simulink model "gm_radarSim4"  (R2023b)
settings: Solver=FixedStepAuto  StartTime=0.0  StopTime=simTime  RelTol=1e-3
libraries: dspsrcs4 x3, dspstat3 x2, paullib x2, simulink x1
settings Model: Creator=pbroo  LastModifiedBy=pbroo
settings SolverCC: AutoInsertRateTranBlk=on
settings OptimizationCC: BlockReduction=off  ConditionallyExecuteInputs=off  DefaultParameterBehavior=Inlined
settings DebuggingCC: AlgebraicLoopMsg=error  InheritedTsInSrcMsg=none  SingleTaskRateTransMsg=error
settings HardwareCC: ProdBitPerPointer=32  ProdBitPerSizeT=32  ProdBitPerPtrDiffT=32  ProdLargestAtomicFloat=None  ProdIntDivRoundTo=Undefined  ProdEndianess=Unspecified  ProdWordSize=32  ProdHWDeviceType=ASIC/FPGA->ASIC/FPGA  TargetBitPerPointer=64  TargetBitPerSizeT=64  TargetBitPerPtrDiffT=64  TargetLongLongMode=on  TargetIntDivRoundTo=Zero  TargetEndianess=LittleEndian  TargetWordSize=64  TargetHWDeviceType=Custom Processor->MATLAB Host Computer  ProdEqTarget=off

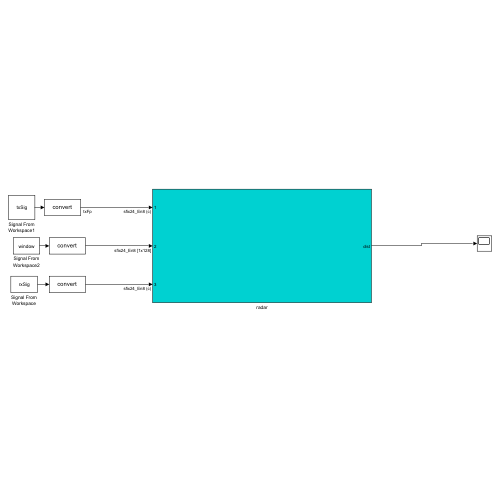
[thumbnail: Simulink's stored preview of the top-level diagram]
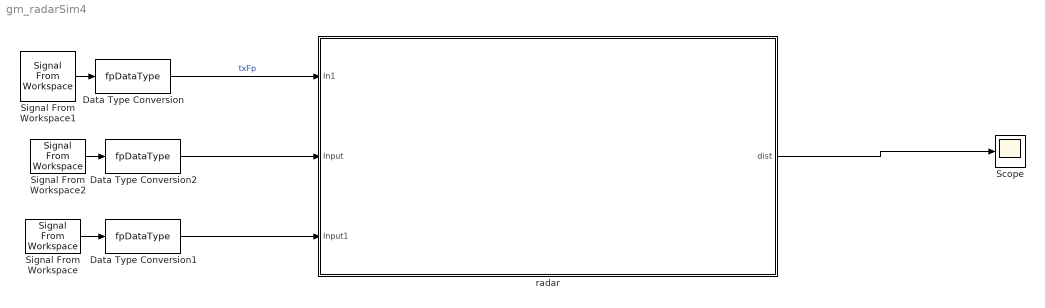
== system gm_radarSim4 ==
  Data Type Conversion : DataTypeConversion  OutDataTypeStr=fpDataType  SaturateOnIntegerOverflow=off  RndMeth=Floor
  Data Type Conversion1 : DataTypeConversion  OutDataTypeStr=fpDataType  SaturateOnIntegerOverflow=off  RndMeth=Floor
  Data Type Conversion2 : DataTypeConversion  OutDataTypeStr=fpDataType  SaturateOnIntegerOverflow=off  RndMeth=Floor
  Scope : Scope
  Signal From Workspace : dspsrcs4/Signal From Workspace  X=rxSig  Ts=1  nsamps=1  OutputAfterFinalValue=Setting to zero  ignoreOrWarnInputAndFrameLengths=off  OutputFrames=off
  Signal From Workspace1 : dspsrcs4/Signal From Workspace  X=txSig  Ts=1  nsamps=1  OutputAfterFinalValue=Setting to zero  ignoreOrWarnInputAndFrameLengths=off  OutputFrames=off
  Signal From Workspace2 : dspsrcs4/Signal From Workspace  X=window  Ts=1  nsamps=1  OutputAfterFinalValue=Setting to zero  ignoreOrWarnInputAndFrameLengths=off  OutputFrames=off
  radar : Subsystem
  wires:
  Data Type Conversion2/1 -> radar/2(Input)
  Signal From Workspace2/1 -> Data Type Conversion2/1
  Data Type Conversion1/1 -> radar/3(Input1)
  Data Type Conversion/1 -> radar/1(In1)  "txFp"
  radar/1(dist) -> Scope/1
  Signal From Workspace/1 -> Data Type Conversion1/1
  Signal From Workspace1/1 -> Data Type Conversion/1

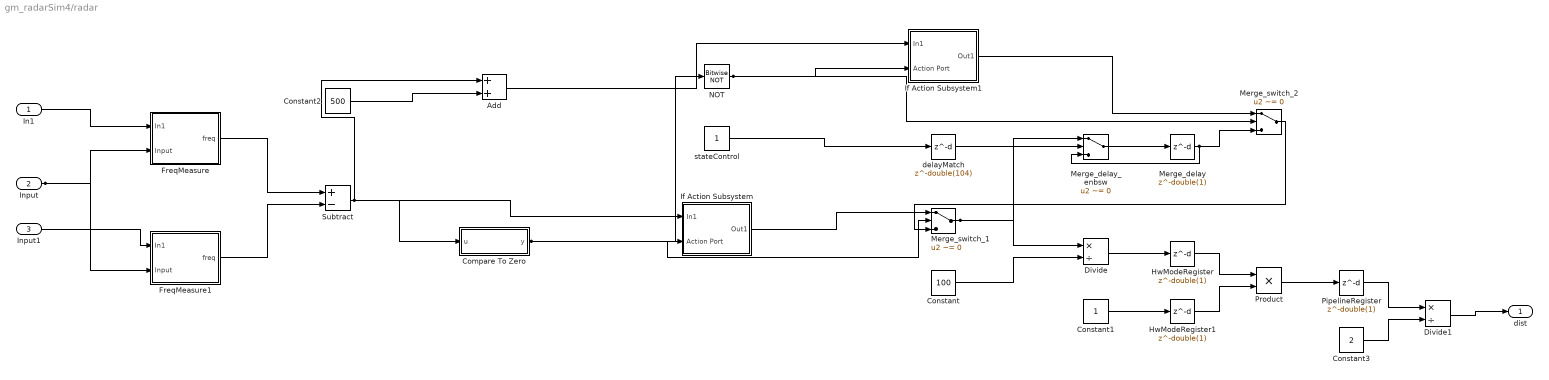
== system gm_radarSim4/radar ==
  In1 : Inport  OutDataTypeStr=fixdt(1, 24, 8)  PortDimensions=1  SampleTime=1
      settings: SignalType=complex
  Input : Inport  Port=2  OutDataTypeStr=fixdt(1, 24, 8)  PortDimensions=[1 128]  SampleTime=1
  Input1 : Inport  Port=3  OutDataTypeStr=fixdt(1, 24, 8)  PortDimensions=1  SampleTime=1
      settings: SignalType=complex
  Add : Sum  OutDataTypeStr=fixdt(1, 24, 8)  AccumDataTypeStr=fixdt(1, 25, 8)  SampleTime=1
  Compare To Zero : Subsystem  mask(Compare To Zero){relop=>=, OutDataTypeStr=boolean, ZeroCross=on}
      mask prompts: relop "Simulink:masks:Operator_MP"; OutDataTypeStr "Simulink:masks:OutputDataType_MP"; ZeroCross "Simulink:masks:EnableZerocrossingDetection_MP"
      mask help: Simulink:masks:CompareToZero_MD
      mask init:
      | OutDataTypeStr = 'boolean';
      | ZeroCross = 'on';
      | blkName = 'radarSim4/radar/Compare\nTo Zero';
      | relop = '>=';
      | setValue = 'boolean';
      mask TypeOptions relop: == | ~= | < | <= | >= | >
      mask TypeOptions OutDataTypeStr: Simulink:masks:uint8 | Simulink:masks:boolean
      mask Callback ZeroCross: sl('zeroCrossEnable', gcbh);
      mask Display: disp([relop,' 0'])
  Constant : Constant  Value=100  OutDataTypeStr=int16  SampleTime=1
  Constant1 : Constant  OutDataTypeStr=int16  SampleTime=1
  Constant2 : Constant  Value=500  OutDataTypeStr=fixdt(1, 24, 8)  SampleTime=1
  Constant3 : Constant  Value=2  VectorParams1D=off  OutDataTypeStr=int16  SampleTime=1
  Divide : Product  Inputs=*/  OutDataTypeStr=fixdt(1, 24, 8)  RndMeth=Simplest  SaturateOnIntegerOverflow=on  SampleTime=1
  Divide1 : Product  Inputs=*/  OutDataTypeStr=fixdt(1, 40, 8)  RndMeth=Simplest  SaturateOnIntegerOverflow=on  SampleTime=1
  FreqMeasure : Subsystem
  FreqMeasure1 : Subsystem
  HwModeRegister : Delay  DelayLength=double(1)  InitialCondition=0  SampleTime=1
  HwModeRegister1 : Delay  DelayLength=double(1)  InitialCondition=0  SampleTime=1
  If Action Subsystem : Subsystem
  If Action Subsystem1 : Subsystem
  Merge_delay : Delay  DelayLength=double(1)  InitialCondition=0  SampleTime=1
  Merge_delay_enbsw : Switch  Criteria=u2 ~= 0  Threshold=double(0)  OutDataTypeStr=fixdt(1, 24, 8)  SampleTime=1  SaturateOnIntegerOverflow=off  InputSameDT=off
  Merge_switch_1 : Switch  Criteria=u2 ~= 0  Threshold=double(0)  OutDataTypeStr=fixdt(1, 24, 8)  SampleTime=1  SaturateOnIntegerOverflow=off  InputSameDT=off
  Merge_switch_2 : Switch  Criteria=u2 ~= 0  Threshold=double(0)  OutDataTypeStr=fixdt(1, 24, 8)  SampleTime=1  SaturateOnIntegerOverflow=off  InputSameDT=off
  NOT : simulink/Logic and Bit Operations/Bitwise Operator  logicop=NOT  UseBitMask=off  BitMask=double(0)  BitMaskRealWorld=Real World Value
  PipelineRegister : Delay  DelayLength=double(1)  InitialCondition=0  SampleTime=1
  Product : Product  Inputs=**  OutDataTypeStr=fixdt(1, 40, 8)  SampleTime=1
  Subtract : Sum  Inputs=+-  OutDataTypeStr=fixdt(1, 24, 8)  AccumDataTypeStr=fixdt(1, 57, 0)  SampleTime=1
  delayMatch : Delay  DelayLength=double(104)  InitialCondition=0  SampleTime=1
  stateControl : Constant  OutDataTypeStr=boolean  SampleTime=1
  dist : Outport  SampleTime=1
  wires:
  In1/1 -> FreqMeasure/1(In1)
  Input/1 -> FreqMeasure1/2(Input), FreqMeasure/2(Input)
  Input1/1 -> FreqMeasure1/1(In1)
  Add/1 -> If Action Subsystem1/1(In1)
  Compare To Zero/1(y) -> NOT/1, If Action Subsystem/2(Action Port), Merge_switch_1/2
  Constant/1 -> Divide/2
  Constant1/1 -> HwModeRegister1/1
  Constant2/1 -> Add/2
  Constant3/1 -> Divide1/2
  Divide/1 -> HwModeRegister/1
  Divide1/1 -> dist/1
  FreqMeasure/1(freq) -> Subtract/1
  FreqMeasure1/1(freq) -> Subtract/2
  PipelineRegister/1 -> Divide1/1
  Subtract/1 -> Add/1, Compare To Zero/1(u), If Action Subsystem/1(In1)
  NOT/1 -> If Action Subsystem1/2(Action Port), Merge_switch_2/2
  stateControl/1 -> delayMatch/1
  Merge_switch_1/1 -> Merge_delay_enbsw/1, Divide/1
  delayMatch/1 -> Merge_delay_enbsw/2
  If Action Subsystem1/1(Out1) -> Merge_switch_2/1
  If Action Subsystem/1(Out1) -> Merge_switch_1/1
  Merge_switch_2/1 -> Merge_switch_1/3
  Merge_delay/1 -> Merge_delay_enbsw/3, Merge_switch_2/3
  Merge_delay_enbsw/1 -> Merge_delay/1
  Product/1 -> PipelineRegister/1
  HwModeRegister/1 -> Product/1
  HwModeRegister1/1 -> Product/2

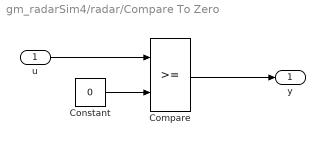
== system gm_radarSim4/radar/Compare To Zero ==
  u : Inport  OutDataTypeStr=fixdt(1, 24, 8)  SampleTime=1
  Compare : RelationalOperator  OutDataTypeStr=boolean
  Constant : Constant  DisableCoverage=on  Value=0  OutDataTypeStr=Inherit: Inherit via back propagation  SampleTime=-1  PreserveConstantTs=on
  y : Outport  SampleTime=1
  wires:
  u/1 -> Compare/1
  Compare/1 -> y/1
  Constant/1 -> Compare/2

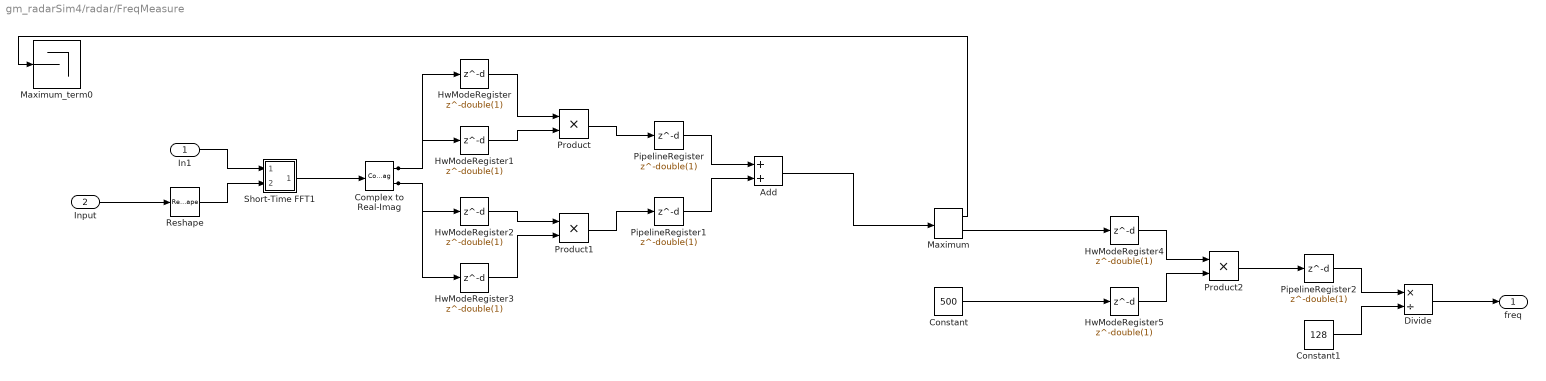
== system gm_radarSim4/radar/FreqMeasure ==
  In1 : Inport  OutDataTypeStr=fixdt(1, 24, 8)  PortDimensions=1  SampleTime=1
      settings: SignalType=complex
  Input : Inport  Port=2  OutDataTypeStr=fixdt(1, 24, 8)  PortDimensions=[1 128]  SampleTime=1
  Add : Sum  OutDataTypeStr=fixdt(1, 63, 16)  AccumDataTypeStr=fixdt(1, 63, 16)  SampleTime=1
  Complex to Real-Imag : ComplexToRealImag  SampleTime=1
  Constant : Constant  Value=500  OutDataTypeStr=fixdt(1, 24, 8)  SampleTime=1
  Constant1 : Constant  Value=128  OutDataTypeStr=fixdt(1, 24, 8)  SampleTime=1
  Divide : Product  Inputs=*/  OutDataTypeStr=fixdt(1, 56, 0)  RndMeth=Simplest  SaturateOnIntegerOverflow=on  SampleTime=1
  HwModeRegister{,1..5} (6 alike) : Delay  DelayLength=double(1)  InitialCondition=0  SampleTime=1
  Maximum : dspstat3/Maximum  operation=maximum  fcn=Value and Index  indexBase=One  operateOver=Each column  Dimension=1  InputProcessing=Columns as channels (frame based)  reset=None  roiEnable=off  roiType=Rectangles  roiPortion=Entire ROI  roiOutput=Individual statistics for each ROI  roiFlag=off  roundingMode=Floor  overflowMode=off  accumDataTypeStr=Inherit: Same as product output  accumLastDataTypeStr=Inherit: Same as product output
  Maximum_term0 : Terminator
  PipelineRegister : Delay  DelayLength=double(1)  InitialCondition=0  SampleTime=1
  PipelineRegister1 : Delay  DelayLength=double(1)  InitialCondition=0  SampleTime=1
  PipelineRegister2 : Delay  DelayLength=double(1)  InitialCondition=0  SampleTime=1
  Product : Product  Inputs=**  OutDataTypeStr=fixdt(1, 62, 16)  SampleTime=1
  Product1 : Product  Inputs=**  OutDataTypeStr=fixdt(1, 62, 16)  SampleTime=1
  Product2 : Product  Inputs=**  OutDataTypeStr=fixdt(1, 56, 8)  SampleTime=1
  Reshape : Reshape  OutputDimensionality=Column vector (2-D)
  Short-Time FFT1 : Subsystem
  freq : Outport  SampleTime=1
  wires:
  In1/1 -> Short-Time FFT1/1(In1)
  Input/1 -> Reshape/1
  Add/1 -> Maximum/1
  Complex to Real-Imag/1 -> HwModeRegister/1, HwModeRegister1/1
  Complex to Real-Imag/2 -> HwModeRegister2/1, HwModeRegister3/1
  Constant/1 -> HwModeRegister5/1
  Constant1/1 -> Divide/2
  Divide/1 -> freq/1
  Maximum/1 -> Maximum_term0/1
  Maximum/2 -> HwModeRegister4/1
  PipelineRegister/1 -> Add/1
  PipelineRegister1/1 -> Add/2
  PipelineRegister2/1 -> Divide/1
  Reshape/1 -> Short-Time FFT1/2(In2)
  Short-Time FFT1/1(Out1) -> Complex to Real-Imag/1
  Product/1 -> PipelineRegister/1
  HwModeRegister/1 -> Product/1
  HwModeRegister1/1 -> Product/2
  Product1/1 -> PipelineRegister1/1
  HwModeRegister2/1 -> Product1/1
  HwModeRegister3/1 -> Product1/2
  Product2/1 -> PipelineRegister2/1
  HwModeRegister4/1 -> Product2/1
  HwModeRegister5/1 -> Product2/2

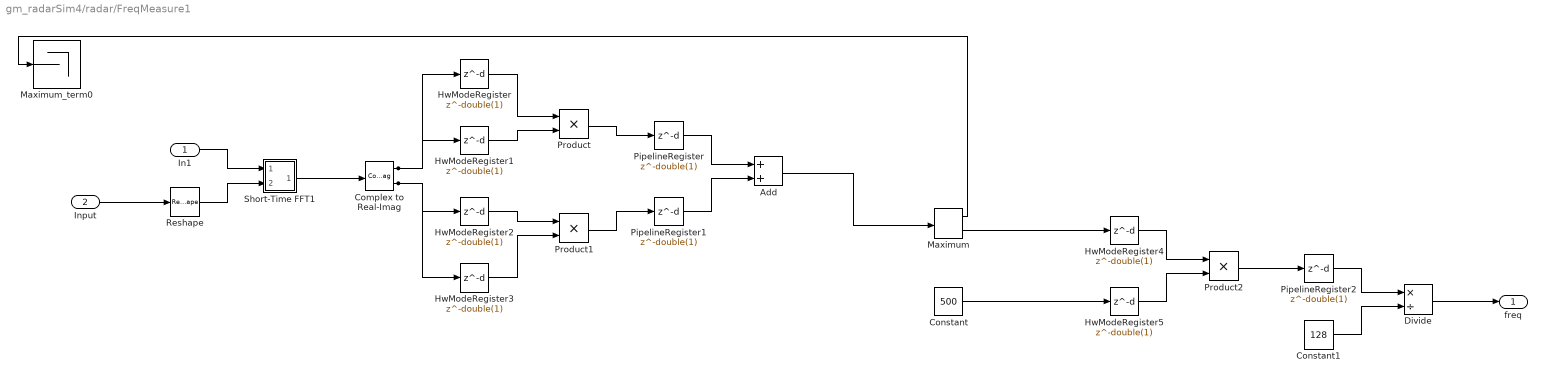
== system gm_radarSim4/radar/FreqMeasure1 ==
  In1 : Inport  OutDataTypeStr=fixdt(1, 24, 8)  PortDimensions=1  SampleTime=1
      settings: SignalType=complex
  Input : Inport  Port=2  OutDataTypeStr=fixdt(1, 24, 8)  PortDimensions=[1 128]  SampleTime=1
  Add : Sum  OutDataTypeStr=fixdt(1, 63, 16)  AccumDataTypeStr=fixdt(1, 63, 16)  SampleTime=1
  Complex to Real-Imag : ComplexToRealImag  SampleTime=1
  Constant : Constant  Value=500  OutDataTypeStr=fixdt(1, 24, 8)  SampleTime=1
  Constant1 : Constant  Value=128  OutDataTypeStr=fixdt(1, 24, 8)  SampleTime=1
  Divide : Product  Inputs=*/  OutDataTypeStr=fixdt(1, 56, 0)  RndMeth=Simplest  SaturateOnIntegerOverflow=on  SampleTime=1
  HwModeRegister{,1..5} (6 alike) : Delay  DelayLength=double(1)  InitialCondition=0  SampleTime=1
  Maximum : dspstat3/Maximum  operation=maximum  fcn=Value and Index  indexBase=One  operateOver=Each column  Dimension=1  InputProcessing=Columns as channels (frame based)  reset=None  roiEnable=off  roiType=Rectangles  roiPortion=Entire ROI  roiOutput=Individual statistics for each ROI  roiFlag=off  roundingMode=Floor  overflowMode=off  accumDataTypeStr=Inherit: Same as product output  accumLastDataTypeStr=Inherit: Same as product output
  Maximum_term0 : Terminator
  PipelineRegister : Delay  DelayLength=double(1)  InitialCondition=0  SampleTime=1
  PipelineRegister1 : Delay  DelayLength=double(1)  InitialCondition=0  SampleTime=1
  PipelineRegister2 : Delay  DelayLength=double(1)  InitialCondition=0  SampleTime=1
  Product : Product  Inputs=**  OutDataTypeStr=fixdt(1, 62, 16)  SampleTime=1
  Product1 : Product  Inputs=**  OutDataTypeStr=fixdt(1, 62, 16)  SampleTime=1
  Product2 : Product  Inputs=**  OutDataTypeStr=fixdt(1, 56, 8)  SampleTime=1
  Reshape : Reshape  OutputDimensionality=Column vector (2-D)
  Short-Time FFT1 : Subsystem
  freq : Outport  SampleTime=1
  wires:
  In1/1 -> Short-Time FFT1/1(In1)
  Input/1 -> Reshape/1
  Add/1 -> Maximum/1
  Complex to Real-Imag/1 -> HwModeRegister/1, HwModeRegister1/1
  Complex to Real-Imag/2 -> HwModeRegister2/1, HwModeRegister3/1
  Constant/1 -> HwModeRegister5/1
  Constant1/1 -> Divide/2
  Divide/1 -> freq/1
  Maximum/1 -> Maximum_term0/1
  Maximum/2 -> HwModeRegister4/1
  PipelineRegister/1 -> Add/1
  PipelineRegister1/1 -> Add/2
  PipelineRegister2/1 -> Divide/1
  Reshape/1 -> Short-Time FFT1/2(In2)
  Short-Time FFT1/1(Out1) -> Complex to Real-Imag/1
  Product/1 -> PipelineRegister/1
  HwModeRegister/1 -> Product/1
  HwModeRegister1/1 -> Product/2
  Product1/1 -> PipelineRegister1/1
  HwModeRegister2/1 -> Product1/1
  HwModeRegister3/1 -> Product1/2
  Product2/1 -> PipelineRegister2/1
  HwModeRegister4/1 -> Product2/1
  HwModeRegister5/1 -> Product2/2

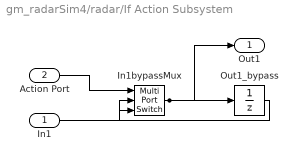
== system gm_radarSim4/radar/If Action Subsystem ==
  In1 : Inport  OutDataTypeStr=fixdt(1, 24, 8)  PortDimensions=1  SampleTime=1
  Action Port : Inport  Port=2  OutDataTypeStr=boolean  SampleTime=1
  In1bypassMux : MultiPortSwitch  DataPortOrder=Zero-based contiguous  Inputs=2  zeroidx=on  OutDataTypeStr=fixdt(1, 24, 8)  SampleTime=1  SaturateOnIntegerOverflow=off  InputSameDT=off
  Out1_bypass : UnitDelay  InitialCondition="fi(0,1,24,8,\"hex\",\"000000\")"  SampleTime=1
  Out1 : Outport  SampleTime=1  InitialOutput=0
  wires:
  In1bypassMux/1 -> Out1/1, Out1_bypass/1
  Action Port/1 -> In1bypassMux/1
  Out1_bypass/1 -> In1bypassMux/2
  In1/1 -> In1bypassMux/3

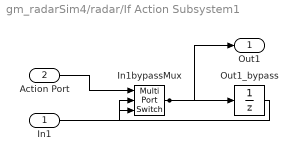
== system gm_radarSim4/radar/If Action Subsystem1 ==
  In1 : Inport  OutDataTypeStr=fixdt(1, 24, 8)  PortDimensions=1  SampleTime=1
  Action Port : Inport  Port=2  OutDataTypeStr=boolean  SampleTime=1
  In1bypassMux : MultiPortSwitch  DataPortOrder=Zero-based contiguous  Inputs=2  zeroidx=on  OutDataTypeStr=fixdt(1, 24, 8)  SampleTime=1  SaturateOnIntegerOverflow=off  InputSameDT=off
  Out1_bypass : UnitDelay  InitialCondition="fi(0,1,24,8,\"hex\",\"000000\")"  SampleTime=1
  Out1 : Outport  SampleTime=1  InitialOutput=0
  wires:
  In1/1 -> In1bypassMux/3
  Out1_bypass/1 -> In1bypassMux/2
  Action Port/1 -> In1bypassMux/1
  In1bypassMux/1 -> Out1_bypass/1, Out1/1

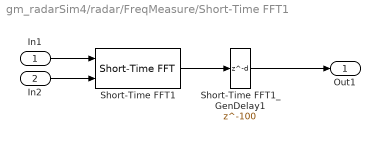
== system gm_radarSim4/radar/FreqMeasure/Short-Time FFT1 ==
  In1 : Inport
  In2 : Inport  Port=2
  Short-Time FFT1 : paullib/Short-Time FFT  W=windowLen  OvLap=nOverlap  M=windowLen
  Short-Time FFT1_GenDelay1 : Delay  DelayLength=100
  Out1 : Outport
  wires:
  In1/1 -> Short-Time FFT1/1
  In2/1 -> Short-Time FFT1/2
  Short-Time FFT1/1 -> Short-Time FFT1_GenDelay1/1
  Short-Time FFT1_GenDelay1/1 -> Out1/1

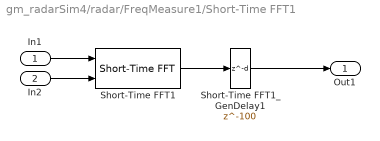
== system gm_radarSim4/radar/FreqMeasure1/Short-Time FFT1 ==
  In1 : Inport
  In2 : Inport  Port=2
  Short-Time FFT1 : paullib/Short-Time FFT  W=windowLen  OvLap=nOverlap  M=windowLen
  Short-Time FFT1_GenDelay1 : Delay  DelayLength=100
  Out1 : Outport
  wires:
  In1/1 -> Short-Time FFT1/1
  In2/1 -> Short-Time FFT1/2
  Short-Time FFT1/1 -> Short-Time FFT1_GenDelay1/1
  Short-Time FFT1_GenDelay1/1 -> Out1/1
